simulink model "Simulink File"  (R2025b)
settings: Solver=VariableStepAuto  StartTime=0.0  StopTime=100  RelTol=1e-3
values from neighbouring files (symbols this model uses):
  A = [-1.064 1.000 ; 290.26 0.00]    [Code.m]
  B = [-0.25 ; -331.40]    [Code.m]
  C = [-123.34 0.00 ; 0.00 1.00]    [Code.m]
  D = [-13.51 ; 0]    [Code.m]
  dT1 = 0.75    [Code.m]
  dT2 = 0.25    [Code.m]
  ELEV_INIT = 10000    [Code.m]
  ELEV_TARGET = 795    [Code.m]
  LAT_OBS = 34.61916    [Code.m]
  LAT_TARGET = 34.6588    [Code.m]
  LON_OBS = -118.8429    [Code.m]
  LON_TARGET = -118.769745    [Code.m]
  Vel = 1021.08    [Code.m]
undefined symbols (not defined in the file or in its folder): K, L
libraries: simulink x3, sensorgpslib x1, slpidlib x1
settings Model: Creator=Pranaya  LastModifiedBy=Pranaya

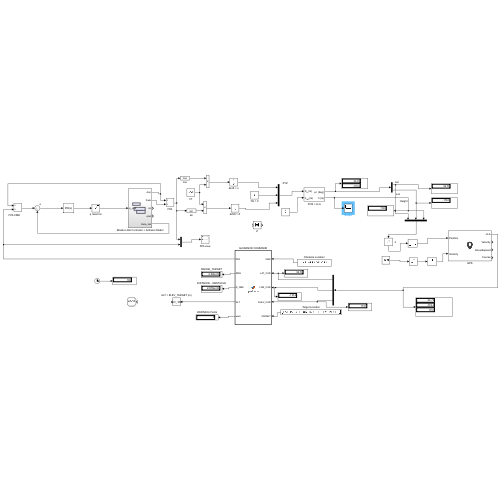
[thumbnail: Simulink's stored preview of the top-level diagram]
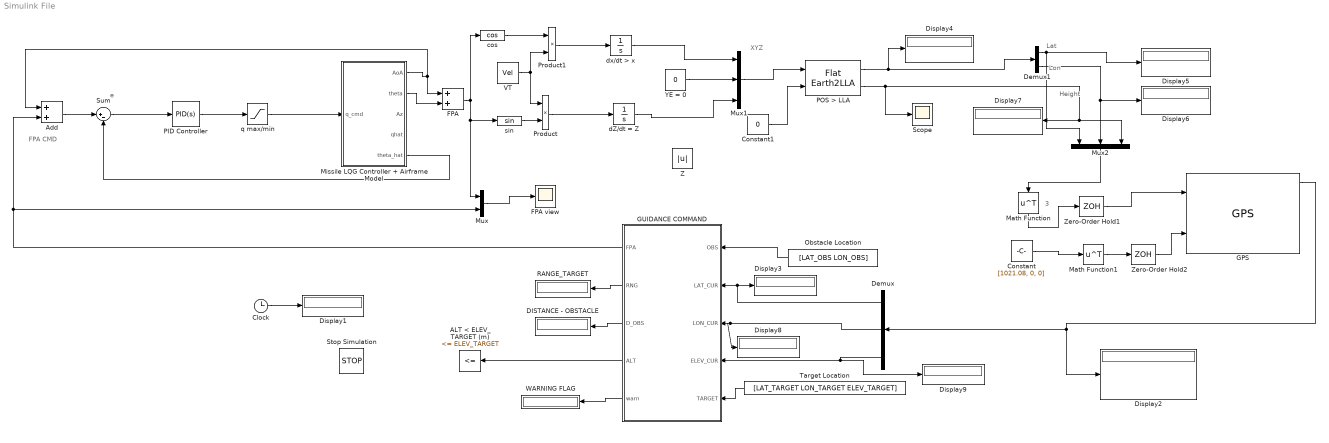
== system Simulink File ==
  note: Height
  note: Lon
  note: Lat
  note: 3
  note: XYZ
  note: FPA CMD
  note: e
  ALT < ELEV_TARGET (m) : simulink/Logic and Bit Operations/Compare To Constant  relop=<=  const=ELEV_TARGET  OutDataTypeStr=boolean
  Add : Sum
  Clock : Clock
  Constant : Constant  Value=[1021.08, 0, 0]
  Constant1 : Constant  Value=0
  DISTANCE - OBSTACLE : Display
  Demux : Demux  Outputs=3
  Demux1 : Demux  Outputs=2
  Display{1..9} (9 alike) : Display
  FPA : Sum
  FPA view : Scope
      settings: ActiveDisplayYMinimum=-0.058305656872177467  ActiveDisplayYMaximum=0.030588765500897751
  GPS : sensorgpslib/GPS  DispRefFrame=NED  PositionInputFormat=Geodetic  ReferenceLocation=[ 0, 0, 0 ]  HorizontalPositionAccuracy=3  VerticalPositionAccuracy=3  VelocityAccuracy=0.1  DecayFactor=0.999  SeedDouble=67  SimulateUsing=Interpreted execution
      settings: LibrarySourceBlock=uavsimlib/GPS
  GUIDANCE COMMAND : MATLAB Function  TreatAsAtomicUnit=on
  Math Function : Math  Operator=transpose
  Math Function1 : Math  Operator=transpose
  Missile LQG Controller + Airframe Model : Subsystem
  Mux : Mux  Inputs=2
  Mux1 : Mux  Inputs=3
  Mux2 : Mux  Inputs=3
  Obstacle Location : Constant  Value=[LAT_OBS LON_OBS]
  PID Controller : slpidlib/PID Controller  Controller=PID  Form=Parallel  TimeDomain=Continuous-time  UseExternalTs=off  SampleTime=-1  IntegratorMethod=Forward Euler  FilterMethod=Forward Euler  ControllerParametersSource=internal  P=-1  I=0  UseKiTs=off  D=0  UseExternalDerivativeSource=off  N=100  UseFilter=on  TunerSelectOption=Transfer Function Based (PID Tuner App)  InitialConditionSource=internal  InitialConditionForIntegrator=0  InitialConditionForFilter=0  DifferentiatorICPrevScaledInput=0  ExternalReset=none  TrackingMode=off  Kt=1  LimitOutput=off  SatLimitsSource=internal  UpperSaturationLimit=inf  LowerSaturationLimit=-inf  LinearizeAsGain=on  AntiWindupMode=none  Kb=1  LimitIntegrator=off  UpperIntegratorSaturationLimit=inf  LowerIntegratorSaturationLimit=-inf  POutMin=[]  POutMax=[]  IOutMin=[]  IOutMax=[]  DOutMin=[]  DOutMax=[]  NOutMin=[]  NOutMax=[]  SumOutMin=[]  SumOutMax=[]  SaturationOutMin=[]  SaturationOutMax=[]  PParamMin=[]  PParamMax=[]  IParamMin=[]  IParamMax=[]  DParamMin=[]  DParamMax=[]  NParamMin=[]  NParamMax=[]  KbParamMin=[]  KbParamMax=[]  KtParamMin=[]  KtParamMax=[]  KbOutMin=[]  KbOutMax=[]  KtOutMin=[]  KtOutMax=[]  IntegratorOutMin=[]  IntegratorOutMax=[]  FilterOutMin=[]  FilterOutMax=[]  SumI1OutMin=[]  SumI1OutMax=[]  SumI2OutMin=[]  SumI2OutMax=[]  SumI3OutMin=[]  SumI3OutMax=[]  SumI4OutMin=[]  SumI4OutMax=[]  SumDOutMin=[]  SumDOutMax=[]  DifferentiatorOutMin=[]  DifferentiatorOutMax=[]  FilterDiffOutCoefMin=[]  FilterDiffOutCoefMax=[]  ReciprocalOutMin=[]  ReciprocalOutMax=[]  SumDenOutMin=[]  SumDenOutMax=[]  SumNumOutMin=[]  SumNumOutMax=[]  DivideOutMin=[]  DivideOutMax=[]  UdiffTsProdOutMin=[]  UdiffTsProdOutMax=[]  NTsProdOutMin=[]  NTsProdOutMax=[]  UintegralTsProdOutMin=[]  UintegralTsProdOutMax=[]  UngainTsProdOutMin=[]  UngainTsProdOutMax=[]  ClampingZeroOutDataTypeStr=Inherit: Inherit via back propagation  ClampingZeroOutMin=[]  ClampingZeroOutMax=[]  FilterDenConstantOutDataTypeStr=Inherit: Inherit via back propagation  FilterDenConstantOutMin=[]  FilterDenConstantOutMax=[]  PCopyOutDataTypeStr=Inherit: Inherit via back propagation  PCopyOutMin=[]  PCopyOutMax=[]  NCopyOutDataTypeStr=Inherit: Inherit via back propagation  NCopyOutMin=[]  NCopyOutMax=[]  IntegratorContinuousStateAttributes=''  IntegratorStateMustResolveToSignalObject=off  IntegratorRTWStateStorageClass=Auto  FilterContinuousStateAttributes=''  FilterStateMustResolveToSignalObject=off  FilterRTWStateStorageClass=Auto  ParallelPVariant=InternalParameters  IdealPVariant=Disabled  IVariant=InternalParameters  DVariant=InternalParameters  IntegratorVariant=Continuous  SatVariant=Disabled  AWVariant=Passthrough  PCopyVariant=Disabled  TRVariant=Disabled  FdbkBlocksVariant=Forward  IdealPFdbkVariant=Disabled  SatFdbkVariant=Disabled  DerivativeFilterVariant=ContFilter  NVariant=InternalParameters  NCopyVariant=Disabled  FilterICVariant=InternalICsFilter  IntegratorICVariant=InternalICs  ExternalResetVariant=Disabled  TRSumVariant=Passthrough  SumFdbkVariant=Disabled  SumVariant=Sum_PID  TsampFilterVariant=InternalTs  TsampNgainVariant=Passthrough  TsampIntegralVariant=Disabled_SignalSpec  ExternalSaturationOutDataTypeStr=Inherit: Same as second input  DerivativeSourceVariant=ErrorSignal  PreIntVariant=InternalPreInt
  POS > LLA : FlatEarth2LLA  LL0=[34.2329 -119.4573]  psi=yaw_init
  Product : Product
  Product1 : Product
  RANGE_TARGET : Display
  Scope : Scope
      settings: ActiveDisplayYMinimum=-274.1851238578854  ActiveDisplayYMaximum=11141.576124873098
  Stop Simulation : Stop
  Sum : Sum  Inputs=|+-
  Target Location : Constant  Value=[LAT_TARGET LON_TARGET ELEV_TARGET]
  VT : Constant  Value=Vel
  WARNING FLAG : Display
  YE = 0 : Constant  Value=0
  Z : Abs  SaturateOnIntegerOverflow=off
  Zero-Order Hold1 : ZeroOrderHold  SampleTime=0.1
  Zero-Order Hold2 : ZeroOrderHold  SampleTime=0.1
  cos : Trigonometry  Operator=cos
  dZ/dt = Z : Integrator  InitialCondition=-ELEV_INIT
  dx/dt > x : Integrator
  q max/min : Saturate
  sin : Trigonometry
  wires:
  Sum/1 -> PID Controller/1
  Missile LQG Controller + Airframe Model/5(theta_hat) -> Sum/2
  Add/1 -> Sum/1
  Missile LQG Controller + Airframe Model/1(AoA) -> Add/1, FPA/1
  Missile LQG Controller + Airframe Model/2(theta) -> FPA/2
  FPA/1 -> cos/1, sin/1, Mux/1
  Mux/1 -> FPA view/1
  VT/1 -> Product/1, Product1/2
  cos/1 -> Product1/1
  sin/1 -> Product/2
  Product1/1 -> dx/dt > x/1
  Product/1 -> dZ/dt = Z/1
  dx/dt > x/1 -> Mux1/1
  YE = 0/1 -> Mux1/2
  Mux1/1 -> POS > LLA/1
  Target Location/1 -> GUIDANCE COMMAND/5(TARGET)
  GUIDANCE COMMAND/4(ALT) -> ALT < ELEV_TARGET (m)/1
  GUIDANCE COMMAND/5(warn) -> WARNING FLAG/1
  GUIDANCE COMMAND/2(RNG) -> RANGE_TARGET/1
  GUIDANCE COMMAND/3(D_OBS) -> DISTANCE - OBSTACLE/1
  GPS/1 -> Demux/1, Display2/1
  Mux2/1 -> Math Function/1
  Constant/1 -> Math Function1/1
  Math Function/1 -> Zero-Order Hold1/1
  Zero-Order Hold1/1 -> GPS/1
  Math Function1/1 -> Zero-Order Hold2/1
  Zero-Order Hold2/1 -> GPS/2
  GUIDANCE COMMAND/1(FPA) -> Mux/2, Add/2
  Clock/1 -> Display1/1
  PID Controller/1 -> q max/min/1
  q max/min/1 -> Missile LQG Controller + Airframe Model/1(q_cmd)
  Obstacle Location/1 -> GUIDANCE COMMAND/1(OBS)
  POS > LLA/1 -> Demux1/1, Display4/1
  Constant1/1 -> POS > LLA/2
  dZ/dt = Z/1 -> Mux1/3
  Demux1/1 -> Display5/1, Mux2/1
  Demux1/2 -> Display6/1, Mux2/2
  POS > LLA/2 -> Scope/1, Display7/1, Mux2/3
  Demux/2 -> Display8/1, GUIDANCE COMMAND/3(LON_CUR)
  Demux/1 -> Display3/1, GUIDANCE COMMAND/2(LAT_CUR)
  Demux/3 -> GUIDANCE COMMAND/4(ELEV_CUR), Display9/1

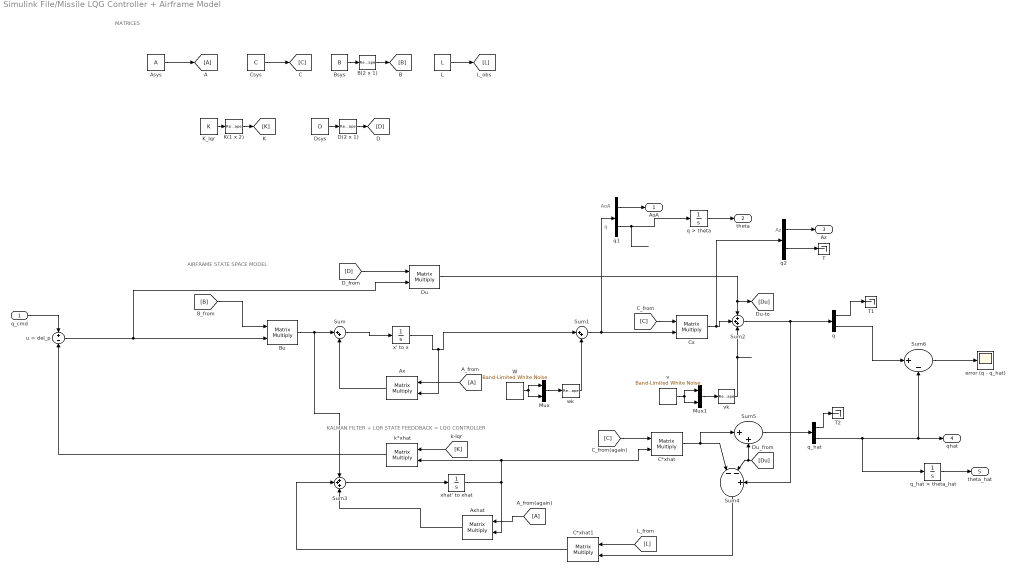
== system Simulink File/Missile LQG Controller + Airframe Model ==
  note: Az
  note: q
  note: AoA
  note: KALMAN FILTER + LQR STATE FEEDDBACK = LQG CONTROLLER
  note: AIRFRAME STATE SPACE MODEL
  note: MATRICES
  q_cmd : Inport
  A : Goto
  A_from : From
  A_from(again) : From
  Asys : Constant  Value=A
  Ax : Product  Multiplication=Matrix(*)
  Axhat : Product  Multiplication=Matrix(*)
  B(2 x 1) : Reshape  OutputDimensionality=Customize  OutputDimensions=[2,1]
  Bsys : Constant  Value=B
  Bu : Product  Multiplication=Matrix(*)
  C*xhat : Product  Multiplication=Matrix(*)
  C*xhat1 : Product  Multiplication=Matrix(*)
  Csys : Constant  Value=C
  Cx : Product  Multiplication=Matrix(*)
  D(2 x 1) : Reshape  OutputDimensionality=Customize  OutputDimensions=[2,1]
  Dsys : Constant  Value=D
  Du : Product  Multiplication=Matrix(*)
  K(1 x 2) : Reshape  OutputDimensionality=Customize  OutputDimensions=[1,2]
  K_lqr : Constant  Value=K
  L : Constant  Value=L
  Mux : Mux  Inputs=2
  Mux1 : Mux  Inputs=2
  Sum : Sum  Inputs=|++
  Sum1 : Sum  Inputs=|++
  Sum2 : Sum  Inputs=+++
  Sum3 : Sum  Inputs=+++
  Sum4 : Sum  Inputs=|--+
  Sum5 : Sum  Inputs=|++
  Sum6 : Sum  Inputs=|+-
  T : Terminator
  T1 : Terminator
  T2 : Terminator
  W : simulink/Sources/Band-Limited White Noise  Cov=[0.00000001]  Ts=dT1  seed=[23341]
  error (q - q_hat) : Scope
      settings: ActiveDisplayYMinimum=-1  ActiveDisplayYMaximum=1
  k*xhat : Product  Multiplication=Matrix(*)
  q : Demux  Outputs=2
  q > theta : Integrator
  q1 : Demux  Outputs=2
  q2 : Demux  Outputs=2
  q_hat : Demux  Outputs=2
  q_hat > theta_hat : Integrator
  u = del_p : Sum  Inputs=+-
  v : simulink/Sources/Band-Limited White Noise  Cov=[0.00001]  Ts=dT2  seed=[23341]
  vk : Reshape  OutputDimensionality=Customize  OutputDimensions=[2,1]
  wk : Reshape  OutputDimensionality=Customize  OutputDimensions=[2,1]
  x' to x : Integrator
  xhat' to xhat : Integrator
  AoA : Outport
  theta : Outport  Port=2
  Az : Outport  Port=3
  qhat : Outport  Port=4
  theta_hat : Outport  Port=5
  wires:
  K_lqr/1 -> K(1 x 2)/1
  Cx/1 -> q2/1, Sum2/2
  Sum/1 -> x' to x/1
  v/1 -> Mux1/2, Mux1/1
  L/1 -> [L]
  q1/2 -> q > theta/1
  xhat' to xhat/1 -> k*xhat/2, C*xhat/2, Axhat/2
  Bsys/1 -> B(2 x 1)/1
  Axhat/1 -> Sum3/3
  Sum6/1 -> error (q - q_hat)/1
  Du/1 -> [Du], Sum2/1
  q1/1 -> AoA/1
  [B] -> Bu/1
  q2/2 -> T/1
  Asys/1 -> A/1
  [D] -> Du/1
  [Du] -> Sum4/2, Sum5/2
  vk/1 -> Sum2/3
  wk/1 -> Sum1/2
  D(2 x 1)/1 -> [D]
  C*xhat/1 -> Sum5/1, Sum4/1
  q_hat/2 -> q_hat > theta_hat/1, qhat/1, Sum6/2
  Ax/1 -> Sum/2
  q/1 -> T1/1
  [C] -> Cx/1
  Csys/1 -> [C]
  C*xhat1/1 -> Sum3/2
  W/1 -> Mux/1, Mux/2
  q_hat/1 -> T2/1
  Bu/1 -> Sum3/1, Sum/1
  K(1 x 2)/1 -> [K]
  Sum1/1 -> q1/1, Cx/2
  [K] -> k*xhat/1
  Sum5/1 -> q_hat/1
  x' to x/1 -> Ax/2, Sum1/1
  Mux1/1 -> vk/1
  q > theta/1 -> theta/1
  Dsys/1 -> D(2 x 1)/1
  u = del_p/1 -> Du/2, Bu/2
  k*xhat/1 -> u = del_p/2
  q/2 -> Sum6/1
  B(2 x 1)/1 -> [B]
  Sum3/1 -> xhat' to xhat/1
  Sum2/1 -> q/1, Sum4/3
  q2/1 -> Az/1
  q_cmd/1 -> u = del_p/1
  Mux/1 -> wk/1
  [C] -> C*xhat/1
  q_hat > theta_hat/1 -> theta_hat/1
  [L] -> C*xhat1/1
  Sum4/1 -> C*xhat1/2
  A_from(again)/1 -> Axhat/1
  A_from/1 -> Ax/1

== matlab function Simulink File/GUIDANCE COMMAND ==
  data: OBS input; FPA output; LAT_CUR input; LON_CUR input; ELEV_CUR input; TARGET input; RNG output; D_OBS output; ALT output; warn output
function [FPA, RNG, D_OBS, ALT, warn] = guidance(OBS, LAT_CUR, LON_CUR, ELEV_CUR, TARGET)
R = 6371000; 
d2r = pi/180;

% OBSTACLE LOCATION
LAT_OBS = OBS(1);
LON_OBS = OBS(2);
thres = 2500; % 2.5km Danger Zone

% TARGET LOCATION
LAT_TARGET = TARGET(1);
LON_TARGET = TARGET(2);
ELEV_TARGET = TARGET(3);

%% distance to target
l1 = LAT_CUR*d2r;
u1 = LON_CUR*d2r;
l2 = LAT_TARGET*d2r;
u2 = LON_TARGET*d2r;

% Current (10000) - Target (795) = +9205m.
dh = ELEV_CUR - ELEV_TARGET; 

dl = l2 - l1;
du = u2 - u1;
a = sin(dl/2)^2 + cos(l1)*cos(l2)*sin(du/2)^2;
c = 2*atan2(sqrt(a),sqrt(1-a));
d = R*c; 

%% distance from the obstacle
l3 = LAT_OBS*d2r;
u3 = LON_OBS*d2r;
dl_obs = l3 - l1;
du_obs = u3 - u1;
a_obs = sin(dl_obs/2)^2 + cos(l1)*cos(l3)*sin(du_obs/2)^2;
c_obs = 2*atan2(sqrt(a_obs),sqrt(1-a_obs));
d_obs = R*c_obs; 

%% current range 
range = sqrt(d^2+dh^2);

%% calculate commanded flight path setpoint
if d_obs >= thres
    w = 0;
    % Positive FPA commands the airframe to DIVE
    FPA_CMD = atan(dh/d); 
else
    w = 1;
    % Negative FPA commands the airframe to CLIMB over the mountain
    FPA_CMD = -0.35; 
end

%% output variables
FPA = FPA_CMD;
RNG = d; 
D_OBS = d_obs;
warn = w;
ALT = ELEV_CUR;
